simulink model "Atomic_Subsystem"  (R2020b)
settings: Solver=FixedStepAuto  StartTime=0.0  StopTime=10.0  FixedStep=0.1  RelTol=1e-3
settings Model: Creator=Puru Gawande  LastModifiedBy=Puru Gawande
settings DataIOCC: SaveOutput=off  SaveTime=off

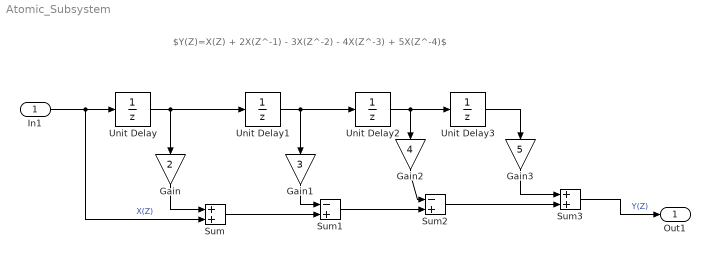
== system Atomic_Subsystem ==
  note: $Y(Z)=X(Z) + 2X(Z^-1) - 3X(Z^-2) - 4X(Z^-3) + 5X(Z^-4)$
  In1 : Inport  OutDataTypeStr=double  PortDimensions=[1 1]  SampleTime=[0.10000000000000001,0]
  Gain : Gain  Gain=2
  Gain1 : Gain  Gain=3
  Gain2 : Gain  Gain=4
  Gain3 : Gain  Gain=5
  Sum : Sum
  Sum1 : Sum  Inputs=-+
  Sum2 : Sum  Inputs=-+
  Sum3 : Sum
  Unit Delay{,1..3} (4 alike) : UnitDelay  SampleTime=-1  HasFrameUpgradeWarning=on
  Out1 : Outport  OutDataTypeStr=double  PortDimensions=[1 1]  SampleTime=[0.10000000000000001,0]
  wires:
  Sum2/1 -> Sum3/2
  Gain3/1 -> Sum3/1
  Sum/1 -> Sum1/2
  Unit Delay3/1 -> Gain3/1
  Gain2/1 -> Sum2/1
  Sum3/1 -> Out1/1  "Y(Z)"
  Gain/1 -> Sum/1
  Gain1/1 -> Sum1/1
  Unit Delay1/1 -> Unit Delay2/1, Gain1/1
  Unit Delay2/1 -> Gain2/1, Unit Delay3/1
  Sum1/1 -> Sum2/2
  Unit Delay/1 -> Unit Delay1/1, Gain/1
  In1/1 -> Sum/2, Unit Delay/1  "X(Z)"
